simulink model "chris_3R_hsv_all_primitives_fixed_vortex"  (R2024b)
settings: Solver=FixedStepDiscrete  StartTime=0.0  StopTime=15  FixedStep=0.1  MaxStep=0.1  RelTol=1e-3
libraries: neural x102, realtime_pacer_lib x1, simulink x1
(part 1 of 6)
settings Model: Creator=RSL  LastModifiedBy=cwaight
settings SolverCC: AlgebraicLoopSolver=TrustRegion
settings DataIOCC: ReturnWorkspaceOutputs=off
settings DebuggingCC: UnconnectedInputMsg=warning  UnconnectedOutputMsg=warning  UnconnectedLineMsg=warning  ArithmeticOperatorsInVariantConditions=warning
settings ModelReferenceCC: EnableRefExpFcnMdlSchedulingChecks=on
settings SFSimCC: SimUseLocalCustomCode=off  CustomCodeUndefinedFunction=UseInterfaceOnly
settings RTWCC: RTWUseLocalCustomCode=off  GPUComputeCapability=3.5
settings CodeAppCC: StateflowObjectComments=on

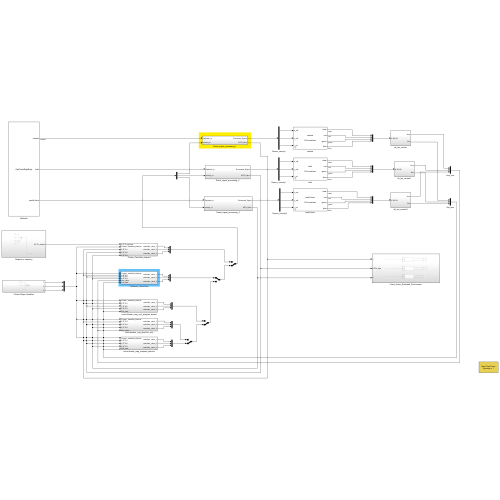
[thumbnail: Simulink's stored preview of the top-level diagram]
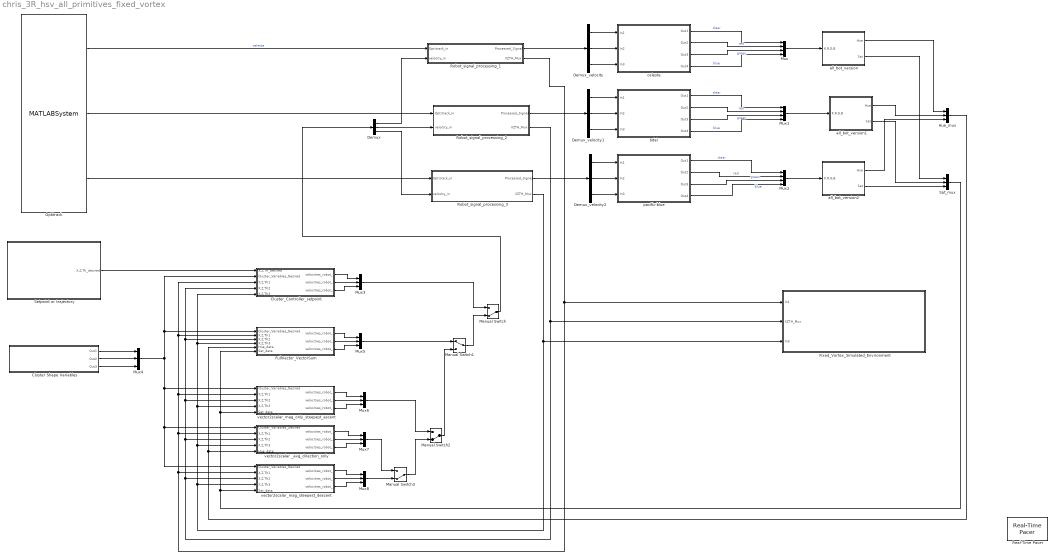
== system chris_3R_hsv_all_primitives_fixed_vortex ==
  Cluster Shape Variables : Subsystem
  Cluster_Controller_setpoint : Subsystem
  Demux : Demux  Outputs=3
  Demux_velocity : Demux  Outputs=3
  Demux_velocity1 : Demux  Outputs=3
  Demux_velocity2 : Demux  Outputs=3
  Fixed_Vortex_Simulated_Environment : Subsystem
  FullVector_VectorSum : Subsystem
  Hue_mux : Mux  Inputs=3
  Manual Switch : ManualSwitch  CurrentSetting=0
  Manual Switch1 : ManualSwitch
  Manual Switch2 : ManualSwitch  CurrentSetting=0
  Manual Switch3 : ManualSwitch  CurrentSetting=0
  Mux : Mux
  Mux1 : Mux
  Mux2 : Mux
  Mux{3..8} (6 alike) : Mux  Inputs=3
  Optitrack : MATLABSystem  System=OptiTrackRigidBody  coordinateTransformationMatrix=[ 1, 0, 0; 0, 0, 1; 0, -1, 0 ]  rigidBodyNames={ 'celeste','tidal','pacific-blue'}  orientationFormat=Euler angles  debug=on  natNetHostAddress=127.0.0.1  natNetClientAddress=127.0.0.1  dllPath=C:\DecaMATLAB\NatNetSDK\lib\x64\NatNetML.dll  unicast=off
      mask Type: OptiTrackRigidBody
      mask Display:
      | disp('OptiTrackRigidBody');
      | port_label('output',1,'celeste');
      | port_label('output',2,'tidal');
      | port_label('output',3,'pacific-blue');
  Real-Time Pacer : realtime_pacer_lib/Real-Time Pacer  simTimePerRealTime=1
  Robot_signal_processing_1 : Subsystem
  Robot_signal_processing_2 : Subsystem
  Robot_signal_processing_3 : Subsystem
  Sat_mux : Mux  Inputs=3
  Setpoint or trajectory : Subsystem
  all_bot_version : Subsystem
  all_bot_version1 : Subsystem
  all_bot_version2 : Subsystem
  celeste : Subsystem  mask(DecabotMask){robotName=celeste, decabotHelper=localhost, robotAddress=, useDataTurbine=off, useDirectSocket=on, debug=off}
      mask prompts: robotName "Robot name:"; decabotHelper "DecabotHelper/DataTurbine server:"; robotAddress "Robot network address (optional):"; useDataTurbine "Use DataTurbine"; useDirectSocket "Use direct robot TCP connection"; debug "Log debug messages"
      mask help: This is a masked subsystem that contains a Decabot block for bidirectional communication with a decabot over a direct TCP socket connection.
      mask init:
      | robotName = 'Nobody';
      | decabotHelper = 'localhost';
      | robotAddress = '';
      | useDataTurbine = true;
      | debug = true;
      mask TypeOptions robotName: decabot/robotName
      mask Callback robotName:
      | try
      |     set_param( gcb( ), 'Name', get_param( gcb( ), 'robotName' ) );
      | end
      mask TypeOptions decabotHelper: decabot/decabotHelper
      mask TypeOptions robotAddress: decabot/robotAddress
      mask TypeOptions useDataTurbine: decabot/useDataTurbine
      mask TypeOptions useDirectSocket: decabot/useDirectSocket
      mask TypeOptions debug: decabot/debug
      mask Display:
      | disp( [get_param( gcb( ), 'robotName' ) '\n\nDH: ' get_param( gcb( ), 'decabotHelper' ) ] );
      | 
      | port_label('input',1,'x_vel');
      | port_label('input',2,'y_vel');
      | port_label('input',3,'t_vel');
      | 
      | port_label('output',1,'clear');
      | port_label('output',2,'red');
      | port_label('output',3,'green');
      | port_label('output',4,'blue');
  pacific-blue : Subsystem  mask(DecabotMask){robotName=pacific-blue, decabotHelper=localhost, robotAddress=, useDataTurbine=off, useDirectSocket=on, debug=off}
      mask prompts: robotName "Robot name:"; decabotHelper "DecabotHelper/DataTurbine server:"; robotAddress "Robot network address (optional):"; useDataTurbine "Use DataTurbine"; useDirectSocket "Use direct robot TCP connection"; debug "Log debug messages"
      mask help: This is a masked subsystem that contains a Decabot block for bidirectional communication with a decabot over a direct TCP socket connection.
      mask init:
      | robotName = 'Nobody';
      | decabotHelper = 'localhost';
      | robotAddress = '';
      | useDataTurbine = true;
      | debug = true;
      mask TypeOptions robotName: decabot/robotName
      mask Callback robotName:
      | try
      |     set_param( gcb( ), 'Name', get_param( gcb( ), 'robotName' ) );
      | end
      mask TypeOptions decabotHelper: decabot/decabotHelper
      mask TypeOptions robotAddress: decabot/robotAddress
      mask TypeOptions useDataTurbine: decabot/useDataTurbine
      mask TypeOptions useDirectSocket: decabot/useDirectSocket
      mask TypeOptions debug: decabot/debug
      mask Display:
      | disp( [get_param( gcb( ), 'robotName' ) '\n\nDH: ' get_param( gcb( ), 'decabotHelper' ) ] );
      | 
      | port_label('input',1,'x_vel');
      | port_label('input',2,'y_vel');
      | port_label('input',3,'t_vel');
      | 
      | port_label('output',1,'clear');
      | port_label('output',2,'red');
      | port_label('output',3,'green');
      | port_label('output',4,'blue');
  tidal : Subsystem  mask(DecabotMask){robotName=tidal, decabotHelper=localhost, robotAddress=, useDataTurbine=off, useDirectSocket=on, debug=off}
      mask prompts: robotName "Robot name:"; decabotHelper "DecabotHelper/DataTurbine server:"; robotAddress "Robot network address (optional):"; useDataTurbine "Use DataTurbine"; useDirectSocket "Use direct robot TCP connection"; debug "Log debug messages"
      mask help: This is a masked subsystem that contains a Decabot block for bidirectional communication with a decabot over a direct TCP socket connection.
      mask init:
      | robotName = 'Nobody';
      | decabotHelper = 'localhost';
      | robotAddress = '';
      | useDataTurbine = true;
      | debug = true;
      mask TypeOptions robotName: decabot/robotName
      mask Callback robotName:
      | try
      |     set_param( gcb( ), 'Name', get_param( gcb( ), 'robotName' ) );
      | end
      mask TypeOptions decabotHelper: decabot/decabotHelper
      mask TypeOptions robotAddress: decabot/robotAddress
      mask TypeOptions useDataTurbine: decabot/useDataTurbine
      mask TypeOptions useDirectSocket: decabot/useDirectSocket
      mask TypeOptions debug: decabot/debug
      mask Display:
      | disp( [get_param( gcb( ), 'robotName' ) '\n\nDH: ' get_param( gcb( ), 'decabotHelper' ) ] );
      | 
      | port_label('input',1,'x_vel');
      | port_label('input',2,'y_vel');
      | port_label('input',3,'t_vel');
      | 
      | port_label('output',1,'clear');
      | port_label('output',2,'red');
      | port_label('output',3,'green');
      | port_label('output',4,'blue');
  vector2scalar _avg_direction_only : Subsystem
  vector2scalar_mag_only_steepest_ascent : Subsystem
  vector2scalar_mag_steepest_descent : Subsystem
  wires:
  Demux_velocity/3 -> celeste/3(In3)
  Demux_velocity/1 -> celeste/1(In1)
  Demux_velocity/2 -> celeste/2(In2)
  Optitrack/1 -> Robot_signal_processing_1/1(Optitrack_in)  "celeste"
  Robot_signal_processing_1/1(Processed_Signal) -> Demux_velocity/1
  celeste/1(Out1) -> Mux/1  "clear"
  celeste/2(Out2) -> Mux/2  "red"
  celeste/3(Out3) -> Mux/3  "green"
  celeste/4(Out4) -> Mux/4  "blue"
  Robot_signal_processing_1/2(XZTH_Mux) -> vector2scalar_mag_steepest_descent/2(X,Z,Th1), vector2scalar _avg_direction_only/2(X,Z,Th1), vector2scalar_mag_only_steepest_ascent/2(X,Z,Th1), FullVector_VectorSum/2(X,Z,Th1), Cluster_Controller_setpoint/3(X,Z,Th1), Fixed_Vortex_Simulated_Environment/1(In1)
  Mux/1 -> all_bot_version/1(K,R,G,B)
  Demux_velocity1/3 -> tidal/3(In3)
  Demux_velocity1/1 -> tidal/1(In1)
  Demux_velocity1/2 -> tidal/2(In2)
  Robot_signal_processing_2/1(Processed_Signal) -> Demux_velocity1/1
  tidal/1(Out1) -> Mux1/1  "clear"
  tidal/2(Out2) -> Mux1/2  "red"
  tidal/3(Out3) -> Mux1/3  "green"
  tidal/4(Out4) -> Mux1/4  "blue"
  Mux1/1 -> all_bot_version1/1(K,R,G,B)
  Demux_velocity2/3 -> pacific-blue/3(In3)
  Demux_velocity2/1 -> pacific-blue/1(In1)
  Demux_velocity2/2 -> pacific-blue/2(In2)
  Robot_signal_processing_3/1(Processed_Signal) -> Demux_velocity2/1
  pacific-blue/1(Out1) -> Mux2/1  "clear"
  pacific-blue/2(Out2) -> Mux2/2  "red"
  pacific-blue/3(Out3) -> Mux2/3  "green"
  pacific-blue/4(Out4) -> Mux2/4  "blue"
  Mux2/1 -> all_bot_version2/1(K,R,G,B)
  Robot_signal_processing_3/2(XZTH_Mux) -> vector2scalar_mag_steepest_descent/4(X,Z,Th3), vector2scalar _avg_direction_only/4(X,Z,Th3), vector2scalar_mag_only_steepest_ascent/4(X,Z,Th3), FullVector_VectorSum/4(X,Z,Th3), Cluster_Controller_setpoint/5(X,Z,Th3), Fixed_Vortex_Simulated_Environment/3(In3)
  Optitrack/2 -> Robot_signal_processing_2/1(Optitrack_in)
  Optitrack/3 -> Robot_signal_processing_3/1(Optitrack_in)
  Cluster_Controller_setpoint/1(velocities_robot_1) -> Mux3/1
  Cluster_Controller_setpoint/3(velocities_robot_3) -> Mux3/3
  Cluster_Controller_setpoint/2(velocities_robot_2) -> Mux3/2
  Mux4/1 -> vector2scalar_mag_only_steepest_ascent/1(Cluster_Variables_Desired), vector2scalar _avg_direction_only/1(Cluster_Variables_Desired), vector2scalar_mag_steepest_descent/1(Cluster_Variables_Desired), FullVector_VectorSum/1(Cluster_Variables_Desired), Cluster_Controller_setpoint/2(Cluster_Variables_Desired)
  Robot_signal_processing_2/2(XZTH_Mux) -> vector2scalar_mag_steepest_descent/3(X,Z,Th2), vector2scalar_mag_only_steepest_ascent/3(X,Z,Th2), FullVector_VectorSum/3(X,Z,Th2), Cluster_Controller_setpoint/4(X,Z,Th2), vector2scalar _avg_direction_only/3(X,Z,Th2), Fixed_Vortex_Simulated_Environment/2(XZTH_Mux)
  Cluster Shape Variables/1(Out1) -> Mux4/1
  Cluster Shape Variables/3(Out3) -> Mux4/3
  Setpoint or trajectory/1(X,Z,Th_desired) -> Cluster_Controller_setpoint/1(X,Z,Th_desired)
  Demux/1 -> Robot_signal_processing_1/2(velocity_in)
  Demux/2 -> Robot_signal_processing_2/2(velocity_in)
  Demux/3 -> Robot_signal_processing_3/2(velocity_in)
  Mux3/1 -> Manual Switch/1
  Manual Switch/1 -> Demux/1
  FullVector_VectorSum/1(velocities_robot_1) -> Mux5/1
  FullVector_VectorSum/2(velocities_robot_2) -> Mux5/2
  FullVector_VectorSum/3(velocities_robot_3) -> Mux5/3
  all_bot_version1/1(Hue) -> Hue_mux/2
  all_bot_version2/1(Hue) -> Hue_mux/3
  all_bot_version2/2(Sat) -> Sat_mux/3
  Hue_mux/1 -> FullVector_VectorSum/5(Hue_data), vector2scalar _avg_direction_only/5(Hue_data)
  Sat_mux/1 -> vector2scalar_mag_steepest_descent/5(Sat_data), FullVector_VectorSum/6(Sat_data), vector2scalar_mag_only_steepest_ascent/5(Sat_data)
  vector2scalar_mag_only_steepest_ascent/1(velocities_robot_1) -> Mux6/1
  vector2scalar_mag_only_steepest_ascent/2(velocities_robot_2) -> Mux6/2
  vector2scalar_mag_only_steepest_ascent/3(velocities_robot_3) -> Mux6/3
  Mux5/1 -> Manual Switch1/1
  Manual Switch1/1 -> Manual Switch/2
  all_bot_version/2(Sat) -> Sat_mux/1
  all_bot_version/1(Hue) -> Hue_mux/1
  Mux6/1 -> Manual Switch2/1
  Manual Switch2/1 -> Manual Switch1/2
  vector2scalar _avg_direction_only/1(velocities_robot_1) -> Mux7/1
  vector2scalar _avg_direction_only/2(velocities_robot_2) -> Mux7/2
  vector2scalar _avg_direction_only/3(velocities_robot_3) -> Mux7/3
  vector2scalar_mag_steepest_descent/3(velocities_robot_3) -> Mux8/3
  vector2scalar_mag_steepest_descent/2(velocities_robot_2) -> Mux8/2
  vector2scalar_mag_steepest_descent/1(velocities_robot_1) -> Mux8/1
  Mux8/1 -> Manual Switch3/2
  Mux7/1 -> Manual Switch3/1
  Manual Switch3/1 -> Manual Switch2/2
  Cluster Shape Variables/2(Out2) -> Mux4/2
  all_bot_version1/2(Sat) -> Sat_mux/2

== system chris_3R_hsv_all_primitives_fixed_vortex/Cluster Shape Variables ==
  Cluster Variable C : Constant  Value=pi/3
  Cluster_Variable_B : Constant  Value=0.35
  Cluster_variable_A : Constant  Value=0.35
  Out1 : Outport
  Out2 : Outport  Port=2
  Out3 : Outport  Port=3
  wires:
  Cluster_variable_A/1 -> Out1/1
  Cluster Variable C/1 -> Out3/1
  Cluster_Variable_B/1 -> Out2/1

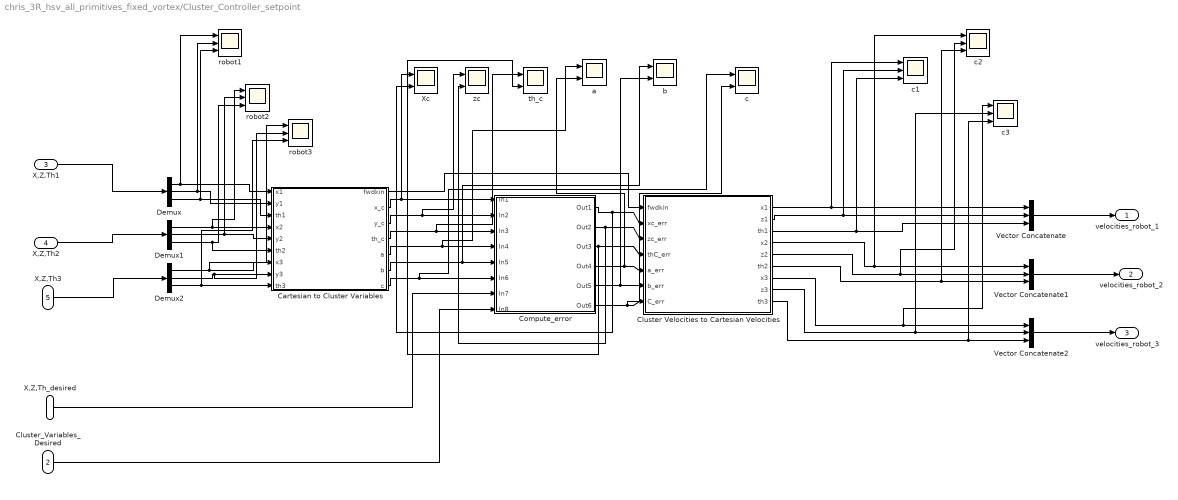
== system chris_3R_hsv_all_primitives_fixed_vortex/Cluster_Controller_setpoint ==
  X,Z,Th_desired : Inport
  Cluster_Variables_Desired : Inport  Port=2
  X,Z,Th1 : Inport  Port=3
  X,Z,Th2 : Inport  Port=4
  X,Z,Th3 : Inport  Port=5
  Cartesian to Cluster Variables : MATLAB Function  TreatAsAtomicUnit=on
  Cluster Velocities to Cartesian Velocities : MATLAB Function  TreatAsAtomicUnit=on
  Compute_error : Subsystem
  Demux : Demux  Outputs=3
  Demux1 : Demux  Outputs=3
  Demux2 : Demux  Outputs=3
  Vector Concatenate : Concatenate  NumInputs=3
  Vector Concatenate1 : Concatenate  NumInputs=3
  Vector Concatenate2 : Concatenate  NumInputs=3
  Xc : Scope  NumInputPorts=2
  a : Scope  NumInputPorts=2
  b : Scope  NumInputPorts=2
  c : Scope  NumInputPorts=2
  c1 : Scope  NumInputPorts=3
  c2 : Scope  NumInputPorts=3
  c3 : Scope  NumInputPorts=3
  robot1 : Scope  NumInputPorts=3
  robot2 : Scope  NumInputPorts=3
  robot3 : Scope  NumInputPorts=3
  th_c : Scope  NumInputPorts=2
  zc : Scope  NumInputPorts=2
  velocities_robot_1 : Outport
  velocities_robot_2 : Outport  Port=2
  velocities_robot_3 : Outport  Port=3
  wires:
  X,Z,Th1/1 -> Demux/1
  X,Z,Th2/1 -> Demux1/1
  X,Z,Th3/1 -> Demux2/1
  Vector Concatenate/1 -> velocities_robot_1/1
  Cluster Velocities to Cartesian Velocities/2(z1) -> c1/2, Vector Concatenate/2
  Cluster Velocities to Cartesian Velocities/1(x1) -> c1/1, Vector Concatenate/1
  Vector Concatenate1/1 -> velocities_robot_2/1
  Cluster Velocities to Cartesian Velocities/5(z2) -> c2/2, Vector Concatenate1/2
  Cluster Velocities to Cartesian Velocities/4(x2) -> c2/1, Vector Concatenate1/1
  Vector Concatenate2/1 -> velocities_robot_3/1
  Cluster Velocities to Cartesian Velocities/8(z3) -> c3/2, Vector Concatenate2/2
  Cluster Velocities to Cartesian Velocities/7(x3) -> c3/1, Vector Concatenate2/1
  Demux/1 -> robot1/1, Cartesian to Cluster Variables/1(x1)
  Demux/2 -> robot1/2, Cartesian to Cluster Variables/2(y1)
  Demux/3 -> robot1/3, Cartesian to Cluster Variables/3(th1)
  Demux1/1 -> robot2/1, Cartesian to Cluster Variables/4(x2)
  Demux1/2 -> robot2/2, Cartesian to Cluster Variables/5(y2)
  Demux1/3 -> robot2/3, Cartesian to Cluster Variables/6(th2)
  Demux2/1 -> robot3/1, Cartesian to Cluster Variables/7(x3)
  Demux2/2 -> robot3/2, Cartesian to Cluster Variables/8(y3)
  Demux2/3 -> robot3/3, Cartesian to Cluster Variables/9(th3)
  Cartesian to Cluster Variables/2(x_c) -> Xc/1, Compute_error/1(In1)
  Cartesian to Cluster Variables/3(y_c) -> zc/1, Compute_error/2(In2)
  Cartesian to Cluster Variables/4(th_c) -> th_c/1, Compute_error/3(In3)
  Cartesian to Cluster Variables/5(a) -> a/1, Compute_error/4(In4)
  Cartesian to Cluster Variables/6(b) -> b/1, Compute_error/5(In5)
  Cartesian to Cluster Variables/7(c) -> c/1, Compute_error/6(In6)
  X,Z,Th_desired/1 -> Compute_error/7(In7)
  Cluster_Variables_Desired/1 -> Compute_error/8(In8)
  Compute_error/1(Out1) -> Xc/2, Cluster Velocities to Cartesian Velocities/2(xc_err)
  Compute_error/2(Out2) -> zc/2, Cluster Velocities to Cartesian Velocities/3(zc_err)
  Compute_error/3(Out3) -> th_c/2, Cluster Velocities to Cartesian Velocities/4(thC_err)
  Compute_error/4(Out4) -> a/2, Cluster Velocities to Cartesian Velocities/5(a_err)
  Compute_error/5(Out5) -> b/2, Cluster Velocities to Cartesian Velocities/6(b_err)
  Compute_error/6(Out6) -> c/2, Cluster Velocities to Cartesian Velocities/7(C_err)
  Cartesian to Cluster Variables/1(fwdkin) -> Cluster Velocities to Cartesian Velocities/1(fwdkin)
  Cluster Velocities to Cartesian Velocities/3(th1) -> c1/3, Vector Concatenate/3
  Cluster Velocities to Cartesian Velocities/6(th2) -> c2/3, Vector Concatenate1/3
  Cluster Velocities to Cartesian Velocities/9(th3) -> c3/3, Vector Concatenate2/3

== system chris_3R_hsv_all_primitives_fixed_vortex/Fixed_Vortex_Simulated_Environment ==
  In1 : Inport
  XZTH_Mux : Inport  Port=2
  In3 : Inport  Port=3
  Demux_velocity1 : Demux  Outputs=3
  Demux_velocity2 : Demux  Outputs=3
  Demux_velocity3 : Demux  Outputs=3
  Fixed_Vortex_Simulator : MATLAB Function  TreatAsAtomicUnit=on
  Fixed_Vortex_Simulator1 : MATLAB Function  TreatAsAtomicUnit=on
  Fixed_Vortex_Simulator2 : MATLAB Function  TreatAsAtomicUnit=on
  To Workspace1 : ToWorkspace  VariableName=hue_anticipated1  SampleTime=-1
  To Workspace2 : ToWorkspace  VariableName=sat_anticipated1  SampleTime=-1
  To Workspace3 : ToWorkspace  VariableName=hue_anticipated2  SampleTime=-1
  To Workspace4 : ToWorkspace  VariableName=sat_anticipated2  SampleTime=-1
  To Workspace5 : ToWorkspace  VariableName=hue_anticipated3  SampleTime=-1
  To Workspace6 : ToWorkspace  VariableName=sat_anticipated3  SampleTime=-1
  wires:
  Demux_velocity3/2 -> Fixed_Vortex_Simulator/2(z)
  Demux_velocity3/3 -> Fixed_Vortex_Simulator/3(th)
  Demux_velocity3/1 -> Fixed_Vortex_Simulator/1(x)
  Fixed_Vortex_Simulator/2(sat_anticipated) -> To Workspace2/1
  Fixed_Vortex_Simulator/1(hue_anticipated) -> To Workspace1/1
  In1/1 -> Demux_velocity3/1
  Fixed_Vortex_Simulator1/1(hue_anticipated) -> To Workspace3/1
  Demux_velocity1/3 -> Fixed_Vortex_Simulator1/3(th)
  Demux_velocity1/1 -> Fixed_Vortex_Simulator1/1(x)
  Fixed_Vortex_Simulator1/2(sat_anticipated) -> To Workspace4/1
  XZTH_Mux/1 -> Demux_velocity1/1
  Demux_velocity1/2 -> Fixed_Vortex_Simulator1/2(z)
  Fixed_Vortex_Simulator2/1(hue_anticipated) -> To Workspace5/1
  Demux_velocity2/3 -> Fixed_Vortex_Simulator2/3(th)
  Demux_velocity2/1 -> Fixed_Vortex_Simulator2/1(x)
  Fixed_Vortex_Simulator2/2(sat_anticipated) -> To Workspace6/1
  In3/1 -> Demux_velocity2/1
  Demux_velocity2/2 -> Fixed_Vortex_Simulator2/2(z)

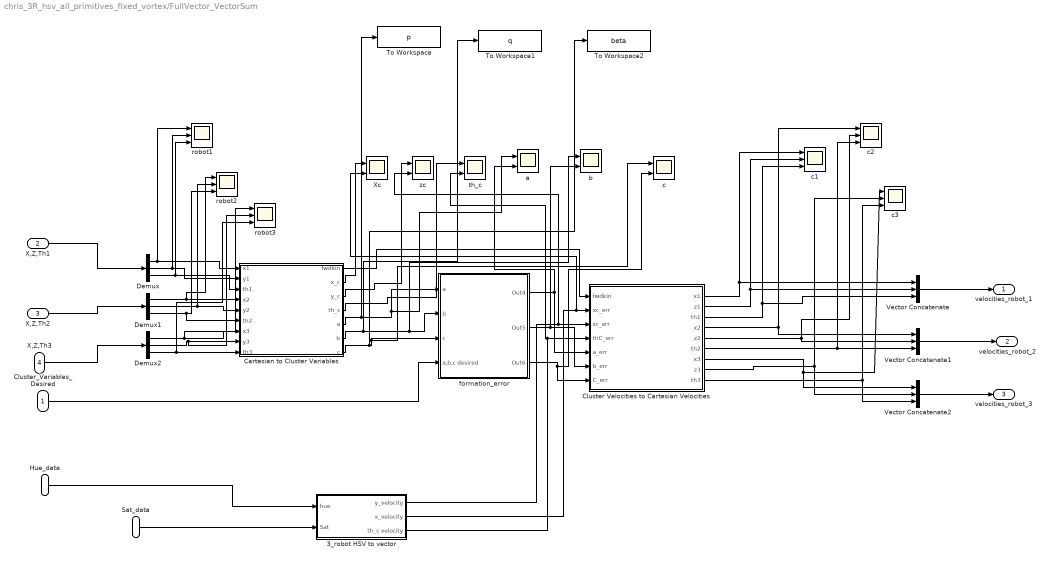
== system chris_3R_hsv_all_primitives_fixed_vortex/FullVector_VectorSum ==
  Cluster_Variables_Desired : Inport
  X,Z,Th1 : Inport  Port=2
  X,Z,Th2 : Inport  Port=3
  X,Z,Th3 : Inport  Port=4
  Hue_data : Inport  Port=5
  Sat_data : Inport  Port=6
  3_robot HSV to vector : Subsystem
  Cartesian to Cluster Variables : MATLAB Function  TreatAsAtomicUnit=on
  Cluster Velocities to Cartesian Velocities : MATLAB Function  TreatAsAtomicUnit=on
  Demux : Demux  Outputs=3
  Demux1 : Demux  Outputs=3
  Demux2 : Demux  Outputs=3
  To Workspace : ToWorkspace  VariableName=p  SampleTime=-1
  To Workspace1 : ToWorkspace  VariableName=q  SampleTime=-1
  To Workspace2 : ToWorkspace  VariableName=beta  SampleTime=-1
  Vector Concatenate : Concatenate  NumInputs=3
  Vector Concatenate1 : Concatenate  NumInputs=3
  Vector Concatenate2 : Concatenate  NumInputs=3
  Xc : Scope  NumInputPorts=2
  a : Scope  NumInputPorts=2
  b : Scope  NumInputPorts=2
  c : Scope  NumInputPorts=2
  c1 : Scope  NumInputPorts=3
  c2 : Scope  NumInputPorts=3
  c3 : Scope  NumInputPorts=3
  formation_error : Subsystem
  robot1 : Scope  NumInputPorts=3
  robot2 : Scope  NumInputPorts=3
  robot3 : Scope  NumInputPorts=3
  th_c : Scope  NumInputPorts=2
  zc : Scope  NumInputPorts=2
  velocities_robot_1 : Outport
  velocities_robot_2 : Outport  Port=2
  velocities_robot_3 : Outport  Port=3
  wires:
  X,Z,Th1/1 -> Demux/1
  X,Z,Th2/1 -> Demux1/1
  X,Z,Th3/1 -> Demux2/1
  Vector Concatenate/1 -> velocities_robot_1/1
  Cluster Velocities to Cartesian Velocities/2(z1) -> c1/2, Vector Concatenate/2
  Cluster Velocities to Cartesian Velocities/1(x1) -> c1/1, Vector Concatenate/1
  Vector Concatenate1/1 -> velocities_robot_2/1
  Cluster Velocities to Cartesian Velocities/5(z2) -> c2/2, Vector Concatenate1/2
  Cluster Velocities to Cartesian Velocities/4(x2) -> c2/1, Vector Concatenate1/1
  Vector Concatenate2/1 -> velocities_robot_3/1
  Cluster Velocities to Cartesian Velocities/8(z3) -> c3/2, Vector Concatenate2/2
  Cluster Velocities to Cartesian Velocities/7(x3) -> Vector Concatenate2/1, c3/1
  Demux/1 -> robot1/1, Cartesian to Cluster Variables/1(x1)
  Demux/2 -> robot1/2, Cartesian to Cluster Variables/2(y1)
  Demux/3 -> robot1/3, Cartesian to Cluster Variables/3(th1)
  Demux1/1 -> robot2/1, Cartesian to Cluster Variables/4(x2)
  Demux1/2 -> robot2/2, Cartesian to Cluster Variables/5(y2)
  Demux1/3 -> robot2/3, Cartesian to Cluster Variables/6(th2)
  Demux2/1 -> robot3/1, Cartesian to Cluster Variables/7(x3)
  Demux2/2 -> robot3/2, Cartesian to Cluster Variables/8(y3)
  Demux2/3 -> robot3/3, Cartesian to Cluster Variables/9(th3)
  Cartesian to Cluster Variables/2(x_c) -> Xc/1
  Cartesian to Cluster Variables/3(y_c) -> zc/1
  Cartesian to Cluster Variables/4(th_c) -> th_c/1
  Cartesian to Cluster Variables/5(a) -> To Workspace/1, a/1, formation_error/1(a)
  Cartesian to Cluster Variables/6(b) -> To Workspace1/1, b/1, formation_error/2(b)
  Cartesian to Cluster Variables/7(c) -> To Workspace2/1, c/1, formation_error/3(c)
  Cluster_Variables_Desired/1 -> formation_error/4(a,b,c desired)
  formation_error/1(Out4) -> a/2, Cluster Velocities to Cartesian Velocities/5(a_err)
  formation_error/2(Out5) -> b/2, Cluster Velocities to Cartesian Velocities/6(b_err)
  formation_error/3(Out6) -> Cluster Velocities to Cartesian Velocities/7(C_err), c/2
  Cartesian to Cluster Variables/1(fwdkin) -> Cluster Velocities to Cartesian Velocities/1(fwdkin)
  Cluster Velocities to Cartesian Velocities/3(th1) -> c1/3, Vector Concatenate/3
  Cluster Velocities to Cartesian Velocities/6(th2) -> c2/3, Vector Concatenate1/3
  Cluster Velocities to Cartesian Velocities/9(th3) -> c3/3, Vector Concatenate2/3
  Hue_data/1 -> 3_robot HSV to vector/1(hue)
  Sat_data/1 -> 3_robot HSV to vector/2(Sat)
  3_robot HSV to vector/2(x_velocity) -> Xc/2, Cluster Velocities to Cartesian Velocities/2(xc_err)
  3_robot HSV to vector/1(y_velocity) -> Cluster Velocities to Cartesian Velocities/3(zc_err), zc/2
  3_robot HSV to vector/3(th_c velocity) -> Cluster Velocities to Cartesian Velocities/4(thC_err), th_c/2

== system chris_3R_hsv_all_primitives_fixed_vortex/Robot_signal_processing_1 ==
  Optitrack_in : Inport
  velocity_in : Inport  Port=2
  Demux4 : Demux  Outputs=3
  Global to Body Velocities : Product  Multiplication=Matrix(*)
  Global to Body Rotation Matrix : MATLAB Function  TreatAsAtomicUnit=on
  Math Function : Math  Operator=transpose  SignedPower=on
  Signal_Reshape : Reshape  OutputDimensions=6
  Signal_Select : Selector  InputPortWidth=6  IndexOptions=Index vector (dialog)  Indices=[1 2 6]  OutputSizes=1
  To Workspace : ToWorkspace  VariableName=robot1_pose  SampleTime=-1
  Processed_Signal : Outport
  XZTH_Mux : Outport  Port=2
  wires:
  Demux4/3 -> Global to Body Rotation Matrix/1(u)  "theta"
  Global to Body Velocities/1 -> Processed_Signal/1
  Signal_Reshape/1 -> Signal_Select/1
  velocity_in/1 -> Global to Body Velocities/2
  Optitrack_in/1 -> Signal_Reshape/1
  Global to Body Rotation Matrix/1(y) -> Math Function/1
  Math Function/1 -> Global to Body Velocities/1
  Signal_Select/1 -> To Workspace/1, XZTH_Mux/1, Demux4/1

== system chris_3R_hsv_all_primitives_fixed_vortex/Robot_signal_processing_2 ==
  Optitrack_in : Inport
  velocity_in : Inport  Port=2
  Demux4 : Demux  Outputs=3
  Global to Body Velocities : Product  Multiplication=Matrix(*)
  Global to Body Rotation Matrix : MATLAB Function  TreatAsAtomicUnit=on
  Math Function : Math  Operator=transpose  SignedPower=on
  Mux : Mux  Inputs=3
  Signal_Reshape : Reshape  OutputDimensions=6
  Signal_Select : Selector  InputPortWidth=6  IndexOptions=Index vector (dialog)  Indices=[1 2 6]  OutputSizes=1
  To Workspace : ToWorkspace  VariableName=robot2_pose  SampleTime=-1
  Processed_Signal : Outport
  XZTH_Mux : Outport  Port=2
  wires:
  Demux4/1 -> Mux/1  "X"
  Demux4/3 -> Mux/3, Global to Body Rotation Matrix/1(u)  "theta"
  Demux4/2 -> Mux/2  "Z"
  Global to Body Velocities/1 -> Processed_Signal/1
  Signal_Reshape/1 -> Signal_Select/1
  velocity_in/1 -> Global to Body Velocities/2
  Optitrack_in/1 -> Signal_Reshape/1
  Global to Body Rotation Matrix/1(y) -> Math Function/1
  Signal_Select/1 -> To Workspace/1, Demux4/1
  Math Function/1 -> Global to Body Velocities/1
  Mux/1 -> XZTH_Mux/1

== system chris_3R_hsv_all_primitives_fixed_vortex/Robot_signal_processing_3 ==
  Optitrack_in : Inport
  velocity_in : Inport  Port=2
  Demux4 : Demux  Outputs=3
  Global to Body Velocities : Product  Multiplication=Matrix(*)
  Global to Body Rotation Matrix : MATLAB Function  TreatAsAtomicUnit=on
  Math Function : Math  Operator=transpose  SignedPower=on
  Mux : Mux  Inputs=3
  Signal_Reshape : Reshape  OutputDimensions=6
  Signal_Select : Selector  InputPortWidth=6  IndexOptions=Index vector (dialog)  Indices=[1 2 6]  OutputSizes=1
  To Workspace : ToWorkspace  VariableName=robot3_pose  SampleTime=-1
  Processed_Signal : Outport
  XZTH_Mux : Outport  Port=2
  wires:
  Demux4/1 -> Mux/1  "X"
  Demux4/3 -> Mux/3, Global to Body Rotation Matrix/1(u)  "theta"
  Demux4/2 -> Mux/2  "Z"
  Global to Body Velocities/1 -> Processed_Signal/1
  Signal_Reshape/1 -> Signal_Select/1
  velocity_in/1 -> Global to Body Velocities/2
  Optitrack_in/1 -> Signal_Reshape/1
  Global to Body Rotation Matrix/1(y) -> Math Function/1
  Signal_Select/1 -> Demux4/1
  Math Function/1 -> Global to Body Velocities/1
  Mux/1 -> To Workspace/1, XZTH_Mux/1

== system chris_3R_hsv_all_primitives_fixed_vortex/Setpoint or trajectory ==
  Manual Switch : ManualSwitch  CurrentSetting=0
  Mux3 : Mux  Inputs=3
  Ramp : simulink/Sources/Ramp  slope=1  start=0  InitialOutput=0.1
  "Theta_Set Point1 " : Constant  Value=0.1
  X_Set Point : Constant  Value=1.5
  Z_Set Point1 : Constant  Value=0.5
  X,Z,Th_desired : Outport
  wires:
  Mux3/1 -> X,Z,Th_desired/1
  Z_Set Point1/1 -> Mux3/2
  Manual Switch/1 -> Mux3/3
  "Theta_Set Point1 "/1 -> Manual Switch/1
  X_Set Point/1 -> Mux3/1
  Ramp/1 -> Manual Switch/2

== system chris_3R_hsv_all_primitives_fixed_vortex/all_bot_version ==
  K,R,G,B : Inport
  Demux : Demux  Outputs=2
  Demux1 : Demux
  Mux : Mux  Inputs=7
  RGB to HSV : MATLAB Function  TreatAsAtomicUnit=on
  everything_hue_net : Subsystem
      mask help: Feed-Forward Neural Network
      mask Display: e = 0.06;c1 = [120 150 230]/255;c2 = ([120 150 230]+0)/383;c3 = ([120 150 230]+128)/383;patch([0 1 1 0],[0 0 1 1],c1);patch([0 1 1 1-e 1-e 0+e],[0 0 1 1-e 0+e 0+e],c2);patch([0 0 1 1-e 0+e 0+e],[0 1 1 1-e 1-e 0+e],c3);plot([0 1 1 0 0],[0 0 1 1 0]);fprintf('NNET');port_label('input',1,' Input');port_label('output',1,'Output ');
  everything_sat_net : Subsystem
      mask help: Feed-Forward Neural Network
      mask Display: e = 0.06;c1 = [120 150 230]/255;c2 = ([120 150 230]+0)/383;c3 = ([120 150 230]+128)/383;patch([0 1 1 0],[0 0 1 1],c1);patch([0 1 1 1-e 1-e 0+e],[0 0 1 1-e 0+e 0+e],c2);patch([0 0 1 1-e 0+e 0+e],[0 1 1 1-e 1-e 0+e],c3);plot([0 1 1 0 0],[0 0 1 1 0]);fprintf('NNET');port_label('input',1,' Input');port_label('output',1,'Output ');
  hue_post_processor : MATLAB Function  TreatAsAtomicUnit=on
  sat_post_processor : MATLAB Function  TreatAsAtomicUnit=on
  sat_post_processor1 : MATLAB Function  TreatAsAtomicUnit=on
  Hue : Outport
  Sat : Outport  Port=2
  wires:
  K,R,G,B/1 -> Demux1/1
  RGB to HSV/2(G) -> Mux/2
  RGB to HSV/6(S) -> Mux/6
  Mux/1 -> sat_post_processor1/1(data_raw)
  sat_post_processor/1(sat) -> Sat/1
  everything_sat_net/1(Output) -> sat_post_processor/1(sat_nn_output)
  Demux/1 -> hue_post_processor/1(hue_nn_sin)
  RGB to HSV/3(B) -> Mux/3
  RGB to HSV/7(V) -> Mux/7
  everything_hue_net/1(Output) -> Demux/1
  Demux/2 -> hue_post_processor/2(hue_nn_cos)
  hue_post_processor/1(hue) -> Hue/1
  RGB to HSV/1(R) -> Mux/1
  RGB to HSV/5(H) -> Mux/5
  RGB to HSV/4(K) -> Mux/4
  sat_post_processor1/1(data) -> everything_sat_net/1(Input), everything_hue_net/1(Input)
  Demux1/1 -> RGB to HSV/4("K ")
  Demux1/2 -> RGB to HSV/1("R ")
  Demux1/3 -> RGB to HSV/2("G ")
  Demux1/4 -> RGB to HSV/3("B ")

== system chris_3R_hsv_all_primitives_fixed_vortex/all_bot_version1 ==
  K,R,G,B : Inport
  Demux : Demux  Outputs=2
  Demux1 : Demux
  Mux : Mux  Inputs=7
  RGB to HSV : MATLAB Function  TreatAsAtomicUnit=on
  everything_hue_net : Subsystem
      mask help: Feed-Forward Neural Network
      mask Display: e = 0.06;c1 = [120 150 230]/255;c2 = ([120 150 230]+0)/383;c3 = ([120 150 230]+128)/383;patch([0 1 1 0],[0 0 1 1],c1);patch([0 1 1 1-e 1-e 0+e],[0 0 1 1-e 0+e 0+e],c2);patch([0 0 1 1-e 0+e 0+e],[0 1 1 1-e 1-e 0+e],c3);plot([0 1 1 0 0],[0 0 1 1 0]);fprintf('NNET');port_label('input',1,' Input');port_label('output',1,'Output ');
  everything_sat_net : Subsystem
      mask help: Feed-Forward Neural Network
      mask Display: e = 0.06;c1 = [120 150 230]/255;c2 = ([120 150 230]+0)/383;c3 = ([120 150 230]+128)/383;patch([0 1 1 0],[0 0 1 1],c1);patch([0 1 1 1-e 1-e 0+e],[0 0 1 1-e 0+e 0+e],c2);patch([0 0 1 1-e 0+e 0+e],[0 1 1 1-e 1-e 0+e],c3);plot([0 1 1 0 0],[0 0 1 1 0]);fprintf('NNET');port_label('input',1,' Input');port_label('output',1,'Output ');
  hue_post_processor : MATLAB Function  TreatAsAtomicUnit=on
  sat_post_processor : MATLAB Function  TreatAsAtomicUnit=on
  sat_post_processor1 : MATLAB Function  TreatAsAtomicUnit=on
  Hue : Outport
  Sat : Outport  Port=2
  wires:
  K,R,G,B/1 -> Demux1/1
  RGB to HSV/2(G) -> Mux/2
  RGB to HSV/6(S) -> Mux/6
  Mux/1 -> sat_post_processor1/1(data_raw)
  sat_post_processor/1(sat) -> Sat/1
  everything_sat_net/1(Output) -> sat_post_processor/1(sat_nn_output)
  Demux/1 -> hue_post_processor/1(hue_nn_sin)
  RGB to HSV/3(B) -> Mux/3
  RGB to HSV/7(V) -> Mux/7
  everything_hue_net/1(Output) -> Demux/1
  Demux/2 -> hue_post_processor/2(hue_nn_cos)
  hue_post_processor/1(hue) -> Hue/1
  RGB to HSV/1(R) -> Mux/1
  RGB to HSV/5(H) -> Mux/5
  RGB to HSV/4(K) -> Mux/4
  sat_post_processor1/1(data) -> everything_sat_net/1(Input), everything_hue_net/1(Input)
  Demux1/1 -> RGB to HSV/4("K ")
  Demux1/2 -> RGB to HSV/1("R ")
  Demux1/3 -> RGB to HSV/2("G ")
  Demux1/4 -> RGB to HSV/3("B ")

== system chris_3R_hsv_all_primitives_fixed_vortex/all_bot_version2 ==
  K,R,G,B : Inport
  Demux : Demux  Outputs=2
  Demux1 : Demux
  Mux : Mux  Inputs=7
  RGB to HSV : MATLAB Function  TreatAsAtomicUnit=on
  everything_hue_net : Subsystem
      mask help: Feed-Forward Neural Network
      mask Display: e = 0.06;c1 = [120 150 230]/255;c2 = ([120 150 230]+0)/383;c3 = ([120 150 230]+128)/383;patch([0 1 1 0],[0 0 1 1],c1);patch([0 1 1 1-e 1-e 0+e],[0 0 1 1-e 0+e 0+e],c2);patch([0 0 1 1-e 0+e 0+e],[0 1 1 1-e 1-e 0+e],c3);plot([0 1 1 0 0],[0 0 1 1 0]);fprintf('NNET');port_label('input',1,' Input');port_label('output',1,'Output ');
  everything_sat_net : Subsystem
      mask help: Feed-Forward Neural Network
      mask Display: e = 0.06;c1 = [120 150 230]/255;c2 = ([120 150 230]+0)/383;c3 = ([120 150 230]+128)/383;patch([0 1 1 0],[0 0 1 1],c1);patch([0 1 1 1-e 1-e 0+e],[0 0 1 1-e 0+e 0+e],c2);patch([0 0 1 1-e 0+e 0+e],[0 1 1 1-e 1-e 0+e],c3);plot([0 1 1 0 0],[0 0 1 1 0]);fprintf('NNET');port_label('input',1,' Input');port_label('output',1,'Output ');
  hue_post_processor : MATLAB Function  TreatAsAtomicUnit=on
  sat_post_processor : MATLAB Function  TreatAsAtomicUnit=on
  sat_post_processor1 : MATLAB Function  TreatAsAtomicUnit=on
  Hue : Outport
  Sat : Outport  Port=2
  wires:
  K,R,G,B/1 -> Demux1/1
  RGB to HSV/2(G) -> Mux/2
  RGB to HSV/6(S) -> Mux/6
  Mux/1 -> sat_post_processor1/1(data_raw)
  sat_post_processor/1(sat) -> Sat/1
  everything_sat_net/1(Output) -> sat_post_processor/1(sat_nn_output)
  Demux/1 -> hue_post_processor/1(hue_nn_sin)
  RGB to HSV/3(B) -> Mux/3
  RGB to HSV/7(V) -> Mux/7
  everything_hue_net/1(Output) -> Demux/1
  Demux/2 -> hue_post_processor/2(hue_nn_cos)
  hue_post_processor/1(hue) -> Hue/1
  RGB to HSV/1(R) -> Mux/1
  RGB to HSV/5(H) -> Mux/5
  RGB to HSV/4(K) -> Mux/4
  sat_post_processor1/1(data) -> everything_sat_net/1(Input), everything_hue_net/1(Input)
  Demux1/1 -> RGB to HSV/4("K ")
  Demux1/2 -> RGB to HSV/1("R ")
  Demux1/3 -> RGB to HSV/2("G ")
  Demux1/4 -> RGB to HSV/3("B ")

== system chris_3R_hsv_all_primitives_fixed_vortex/celeste ==
  In1 : Inport
  In2 : Inport  Port=2
  In3 : Inport  Port=3
  Signal Specification : SignalSpecification  OutDataTypeStr=double  Dimensions=1
  Signal Specification1 : SignalSpecification  OutDataTypeStr=double  Dimensions=1
  Signal Specification2 : SignalSpecification  OutDataTypeStr=double  Dimensions=1
  decabot : MATLABSystem  System=Decabot  robotName=celeste  decabotHelper=localhost  useDataTurbine=off  useDirectSocket=on  debug=off
      mask Type: Decabot
      mask Display:
      | disp('celeste\n\nDH: localhost');
      | port_label('input',1,'x_vel');
      | port_label('input',2,'y_vel');
      | port_label('input',3,'t_vel');
      | port_label('output',1,'clear');
      | port_label('output',2,'red');
      | port_label('output',3,'green');
      | port_label('output',4,'blue');
  Out1 : Outport
  Out2 : Outport  Port=2
  Out3 : Outport  Port=3
  Out4 : Outport  Port=4
  wires:
  Signal Specification2/1 -> decabot/3
  Signal Specification1/1 -> decabot/2
  Signal Specification/1 -> decabot/1
  In2/1 -> Signal Specification1/1
  decabot/4 -> Out4/1
  decabot/1 -> Out1/1
  decabot/3 -> Out3/1
  decabot/2 -> Out2/1
  In1/1 -> Signal Specification/1
  In3/1 -> Signal Specification2/1

== system chris_3R_hsv_all_primitives_fixed_vortex/pacific-blue ==
  In1 : Inport
  In2 : Inport  Port=2
  In3 : Inport  Port=3
  Signal Specification : SignalSpecification  OutDataTypeStr=double  Dimensions=1
  Signal Specification1 : SignalSpecification  OutDataTypeStr=double  Dimensions=1
  Signal Specification2 : SignalSpecification  OutDataTypeStr=double  Dimensions=1
  decabot : MATLABSystem  System=Decabot  robotName=pacific-blue  decabotHelper=localhost  useDataTurbine=off  useDirectSocket=on  debug=off
      mask Type: Decabot
      mask Display:
      | disp('pacific-blue\n\nDH: localhost');
      | port_label('input',1,'x_vel');
      | port_label('input',2,'y_vel');
      | port_label('input',3,'t_vel');
      | port_label('output',1,'clear');
      | port_label('output',2,'red');
      | port_label('output',3,'green');
      | port_label('output',4,'blue');
  Out1 : Outport
  Out2 : Outport  Port=2
  Out3 : Outport  Port=3
  Out4 : Outport  Port=4
  wires:
  Signal Specification2/1 -> decabot/3
  Signal Specification1/1 -> decabot/2
  Signal Specification/1 -> decabot/1
  In2/1 -> Signal Specification1/1
  decabot/4 -> Out4/1
  decabot/1 -> Out1/1
  decabot/3 -> Out3/1
  decabot/2 -> Out2/1
  In1/1 -> Signal Specification/1
  In3/1 -> Signal Specification2/1

== system chris_3R_hsv_all_primitives_fixed_vortex/tidal ==
  In1 : Inport
  In2 : Inport  Port=2
  In3 : Inport  Port=3
  Signal Specification : SignalSpecification  OutDataTypeStr=double  Dimensions=1
  Signal Specification1 : SignalSpecification  OutDataTypeStr=double  Dimensions=1
  Signal Specification2 : SignalSpecification  OutDataTypeStr=double  Dimensions=1
  decabot : MATLABSystem  System=Decabot  robotName=tidal  decabotHelper=localhost  useDataTurbine=off  useDirectSocket=on  debug=off
      mask Type: Decabot
      mask Display:
      | disp('tidal\n\nDH: localhost');
      | port_label('input',1,'x_vel');
      | port_label('input',2,'y_vel');
      | port_label('input',3,'t_vel');
      | port_label('output',1,'clear');
      | port_label('output',2,'red');
      | port_label('output',3,'green');
      | port_label('output',4,'blue');
  Out1 : Outport
  Out2 : Outport  Port=2
  Out3 : Outport  Port=3
  Out4 : Outport  Port=4
  wires:
  Signal Specification2/1 -> decabot/3
  Signal Specification1/1 -> decabot/2
  Signal Specification/1 -> decabot/1
  In2/1 -> Signal Specification1/1
  decabot/4 -> Out4/1
  decabot/1 -> Out1/1
  decabot/3 -> Out3/1
  decabot/2 -> Out2/1
  In1/1 -> Signal Specification/1
  In3/1 -> Signal Specification2/1

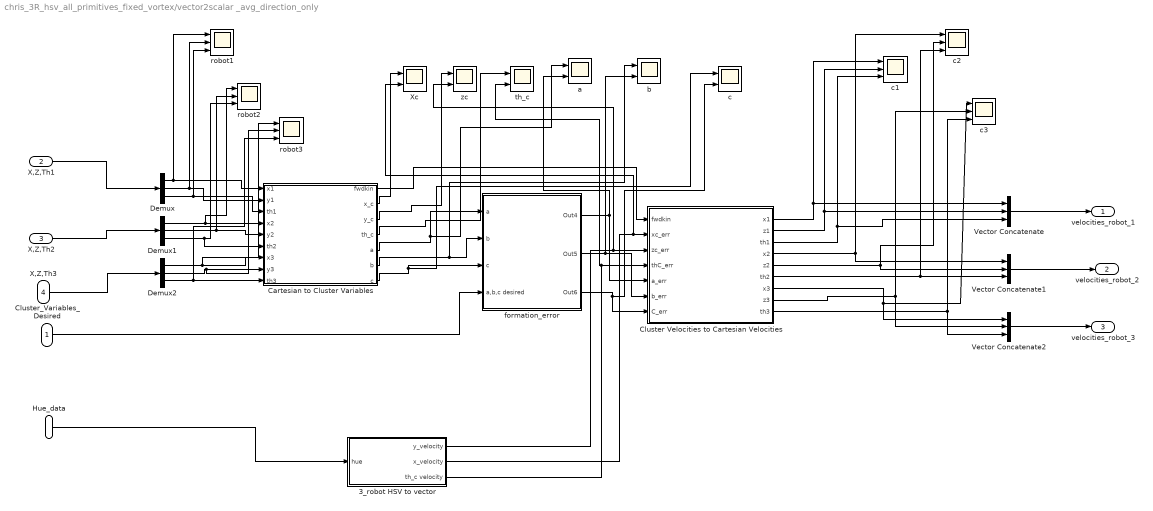
== system chris_3R_hsv_all_primitives_fixed_vortex/vector2scalar _avg_direction_only ==
  Cluster_Variables_Desired : Inport
  X,Z,Th1 : Inport  Port=2
  X,Z,Th2 : Inport  Port=3
  X,Z,Th3 : Inport  Port=4
  Hue_data : Inport  Port=5
  3_robot HSV to vector : Subsystem
  Cartesian to Cluster Variables : MATLAB Function  TreatAsAtomicUnit=on
  Cluster Velocities to Cartesian Velocities : MATLAB Function  TreatAsAtomicUnit=on
  Demux : Demux  Outputs=3
  Demux1 : Demux  Outputs=3
  Demux2 : Demux  Outputs=3
  Vector Concatenate : Concatenate  NumInputs=3
  Vector Concatenate1 : Concatenate  NumInputs=3
  Vector Concatenate2 : Concatenate  NumInputs=3
  Xc : Scope  NumInputPorts=2
  a : Scope  NumInputPorts=2
  b : Scope  NumInputPorts=2
  c : Scope  NumInputPorts=2
  c1 : Scope  NumInputPorts=3
  c2 : Scope  NumInputPorts=3
  c3 : Scope  NumInputPorts=3
  formation_error : Subsystem
  robot1 : Scope  NumInputPorts=3
  robot2 : Scope  NumInputPorts=3
  robot3 : Scope  NumInputPorts=3
  th_c : Scope  NumInputPorts=2
  zc : Scope  NumInputPorts=2
  velocities_robot_1 : Outport
  velocities_robot_2 : Outport  Port=2
  velocities_robot_3 : Outport  Port=3
  wires:
  X,Z,Th1/1 -> Demux/1
  X,Z,Th2/1 -> Demux1/1
  X,Z,Th3/1 -> Demux2/1
  Vector Concatenate/1 -> velocities_robot_1/1
  Cluster Velocities to Cartesian Velocities/2(z1) -> c1/2, Vector Concatenate/2
  Cluster Velocities to Cartesian Velocities/1(x1) -> c1/1, Vector Concatenate/1
  Vector Concatenate1/1 -> velocities_robot_2/1
  Cluster Velocities to Cartesian Velocities/5(z2) -> c2/2, Vector Concatenate1/2
  Cluster Velocities to Cartesian Velocities/4(x2) -> c2/1, Vector Concatenate1/1
  Vector Concatenate2/1 -> velocities_robot_3/1
  Cluster Velocities to Cartesian Velocities/8(z3) -> c3/2, Vector Concatenate2/2
  Cluster Velocities to Cartesian Velocities/7(x3) -> Vector Concatenate2/1, c3/1
  Demux/1 -> robot1/1, Cartesian to Cluster Variables/1(x1)
  Demux/2 -> robot1/2, Cartesian to Cluster Variables/2(y1)
  Demux/3 -> robot1/3, Cartesian to Cluster Variables/3(th1)
  Demux1/1 -> robot2/1, Cartesian to Cluster Variables/4(x2)
  Demux1/2 -> robot2/2, Cartesian to Cluster Variables/5(y2)
  Demux1/3 -> robot2/3, Cartesian to Cluster Variables/6(th2)
  Demux2/1 -> robot3/1, Cartesian to Cluster Variables/7(x3)
  Demux2/2 -> robot3/2, Cartesian to Cluster Variables/8(y3)
  Demux2/3 -> robot3/3, Cartesian to Cluster Variables/9(th3)
  Cartesian to Cluster Variables/2(x_c) -> Xc/1
  Cartesian to Cluster Variables/3(y_c) -> zc/1
  Cartesian to Cluster Variables/4(th_c) -> th_c/1
  Cartesian to Cluster Variables/5(a) -> a/1, formation_error/1(a)
  Cartesian to Cluster Variables/6(b) -> b/1, formation_error/2(b)
  Cartesian to Cluster Variables/7(c) -> c/1, formation_error/3(c)
  Cluster_Variables_Desired/1 -> formation_error/4(a,b,c desired)
  formation_error/1(Out4) -> a/2, Cluster Velocities to Cartesian Velocities/5(a_err)
  formation_error/2(Out5) -> b/2, Cluster Velocities to Cartesian Velocities/6(b_err)
  formation_error/3(Out6) -> Cluster Velocities to Cartesian Velocities/7(C_err), c/2
  Cartesian to Cluster Variables/1(fwdkin) -> Cluster Velocities to Cartesian Velocities/1(fwdkin)
  Cluster Velocities to Cartesian Velocities/3(th1) -> c1/3, Vector Concatenate/3
  Cluster Velocities to Cartesian Velocities/6(th2) -> c2/3, Vector Concatenate1/3
  Cluster Velocities to Cartesian Velocities/9(th3) -> c3/3, Vector Concatenate2/3
  Hue_data/1 -> 3_robot HSV to vector/1(hue)
  3_robot HSV to vector/2(x_velocity) -> Xc/2, Cluster Velocities to Cartesian Velocities/2(xc_err)
  3_robot HSV to vector/1(y_velocity) -> Cluster Velocities to Cartesian Velocities/3(zc_err), zc/2
  3_robot HSV to vector/3(th_c velocity) -> Cluster Velocities to Cartesian Velocities/4(thC_err), th_c/2

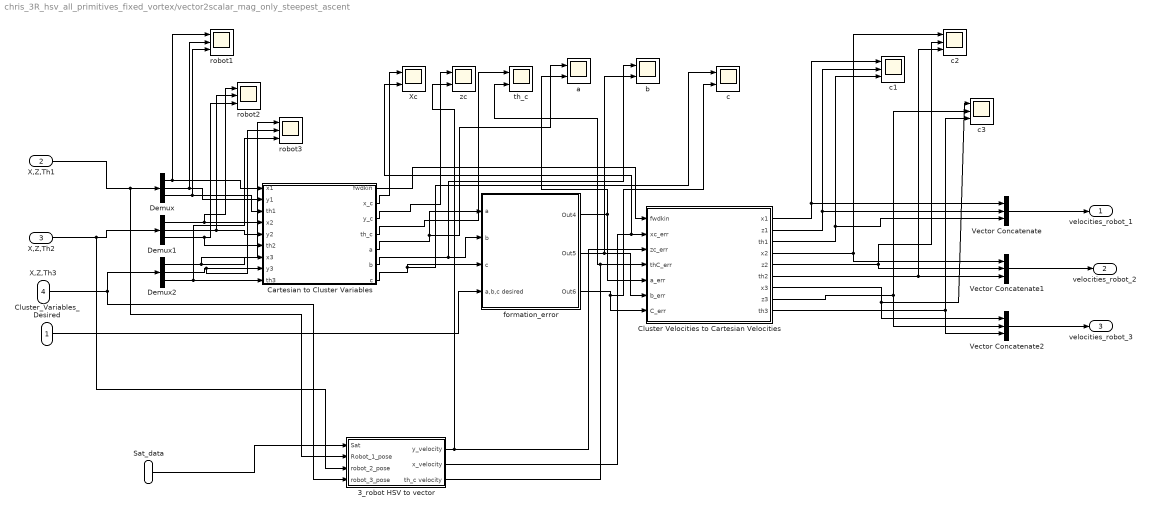
== system chris_3R_hsv_all_primitives_fixed_vortex/vector2scalar_mag_only_steepest_ascent ==
  Cluster_Variables_Desired : Inport
  X,Z,Th1 : Inport  Port=2
  X,Z,Th2 : Inport  Port=3
  X,Z,Th3 : Inport  Port=4
  Sat_data : Inport  Port=5
  3_robot HSV to vector : Subsystem
  Cartesian to Cluster Variables : MATLAB Function  TreatAsAtomicUnit=on
  Cluster Velocities to Cartesian Velocities : MATLAB Function  TreatAsAtomicUnit=on
  Demux : Demux  Outputs=3
  Demux1 : Demux  Outputs=3
  Demux2 : Demux  Outputs=3
  Vector Concatenate : Concatenate  NumInputs=3
  Vector Concatenate1 : Concatenate  NumInputs=3
  Vector Concatenate2 : Concatenate  NumInputs=3
  Xc : Scope  NumInputPorts=2
  a : Scope  NumInputPorts=2
  b : Scope  NumInputPorts=2
  c : Scope  NumInputPorts=2
  c1 : Scope  NumInputPorts=3
  c2 : Scope  NumInputPorts=3
  c3 : Scope  NumInputPorts=3
  formation_error : Subsystem
  robot1 : Scope  NumInputPorts=3
  robot2 : Scope  NumInputPorts=3
  robot3 : Scope  NumInputPorts=3
  th_c : Scope  NumInputPorts=2
  zc : Scope  NumInputPorts=2
  velocities_robot_1 : Outport
  velocities_robot_2 : Outport  Port=2
  velocities_robot_3 : Outport  Port=3
  wires:
  X,Z,Th1/1 -> 3_robot HSV to vector/2(Robot_1_pose), Demux/1
  X,Z,Th2/1 -> 3_robot HSV to vector/3(robot_2_pose), Demux1/1
  X,Z,Th3/1 -> Demux2/1, 3_robot HSV to vector/4(robot_3_pose)
  Vector Concatenate/1 -> velocities_robot_1/1
  Cluster Velocities to Cartesian Velocities/2(z1) -> c1/2, Vector Concatenate/2
  Cluster Velocities to Cartesian Velocities/1(x1) -> c1/1, Vector Concatenate/1
  Vector Concatenate1/1 -> velocities_robot_2/1
  Cluster Velocities to Cartesian Velocities/5(z2) -> c2/2, Vector Concatenate1/2
  Cluster Velocities to Cartesian Velocities/4(x2) -> c2/1, Vector Concatenate1/1
  Vector Concatenate2/1 -> velocities_robot_3/1
  Cluster Velocities to Cartesian Velocities/8(z3) -> c3/2, Vector Concatenate2/2
  Cluster Velocities to Cartesian Velocities/7(x3) -> Vector Concatenate2/1, c3/1
  Demux/1 -> robot1/1, Cartesian to Cluster Variables/1(x1)
  Demux/2 -> robot1/2, Cartesian to Cluster Variables/2(y1)
  Demux/3 -> robot1/3, Cartesian to Cluster Variables/3(th1)
  Demux1/1 -> robot2/1, Cartesian to Cluster Variables/4(x2)
  Demux1/2 -> robot2/2, Cartesian to Cluster Variables/5(y2)
  Demux1/3 -> robot2/3, Cartesian to Cluster Variables/6(th2)
  Demux2/1 -> robot3/1, Cartesian to Cluster Variables/7(x3)
  Demux2/2 -> robot3/2, Cartesian to Cluster Variables/8(y3)
  Demux2/3 -> robot3/3, Cartesian to Cluster Variables/9(th3)
  Cartesian to Cluster Variables/2(x_c) -> Xc/1
  Cartesian to Cluster Variables/3(y_c) -> zc/1
  Cartesian to Cluster Variables/4(th_c) -> th_c/1
  Cartesian to Cluster Variables/5(a) -> a/1, formation_error/1(a)
  Cartesian to Cluster Variables/6(b) -> b/1, formation_error/2(b)
  Cartesian to Cluster Variables/7(c) -> c/1, formation_error/3(c)
  Cluster_Variables_Desired/1 -> formation_error/4(a,b,c desired)
  formation_error/1(Out4) -> a/2, Cluster Velocities to Cartesian Velocities/5(a_err)
  formation_error/2(Out5) -> b/2, Cluster Velocities to Cartesian Velocities/6(b_err)
  formation_error/3(Out6) -> Cluster Velocities to Cartesian Velocities/7(C_err), c/2
  Cartesian to Cluster Variables/1(fwdkin) -> Cluster Velocities to Cartesian Velocities/1(fwdkin)
  Cluster Velocities to Cartesian Velocities/3(th1) -> c1/3, Vector Concatenate/3
  Cluster Velocities to Cartesian Velocities/6(th2) -> c2/3, Vector Concatenate1/3
  Cluster Velocities to Cartesian Velocities/9(th3) -> c3/3, Vector Concatenate2/3
  Sat_data/1 -> 3_robot HSV to vector/1(Sat)
  3_robot HSV to vector/2(x_velocity) -> Xc/2, Cluster Velocities to Cartesian Velocities/2(xc_err)
  3_robot HSV to vector/1(y_velocity) -> Cluster Velocities to Cartesian Velocities/3(zc_err), zc/2
  3_robot HSV to vector/3(th_c velocity) -> Cluster Velocities to Cartesian Velocities/4(thC_err), th_c/2

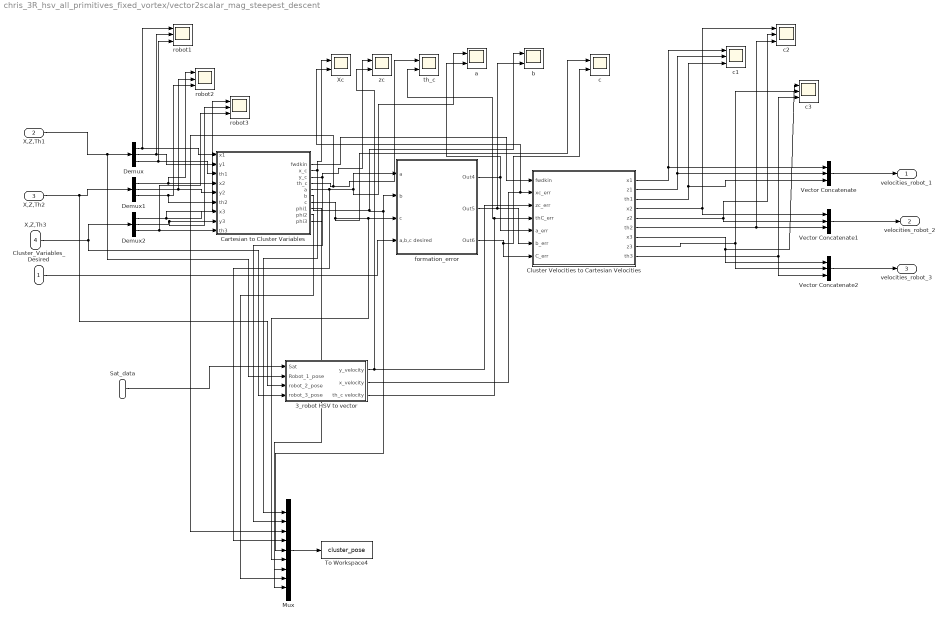
== system chris_3R_hsv_all_primitives_fixed_vortex/vector2scalar_mag_steepest_descent ==
  Cluster_Variables_Desired : Inport
  X,Z,Th1 : Inport  Port=2
  X,Z,Th2 : Inport  Port=3
  X,Z,Th3 : Inport  Port=4
  Sat_data : Inport  Port=5
  3_robot HSV to vector : Subsystem
  Cartesian to Cluster Variables : MATLAB Function  TreatAsAtomicUnit=on
  Cluster Velocities to Cartesian Velocities : MATLAB Function  TreatAsAtomicUnit=on
  Demux : Demux  Outputs=3
  Demux1 : Demux  Outputs=3
  Demux2 : Demux  Outputs=3
  Mux : Mux  Inputs=9
  To Workspace4 : ToWorkspace  VariableName=cluster_pose  SampleTime=-1
  Vector Concatenate : Concatenate  NumInputs=3
  Vector Concatenate1 : Concatenate  NumInputs=3
  Vector Concatenate2 : Concatenate  NumInputs=3
  Xc : Scope  NumInputPorts=2
  a : Scope  NumInputPorts=2
  b : Scope  NumInputPorts=2
  c : Scope  NumInputPorts=2
  c1 : Scope  NumInputPorts=3
  c2 : Scope  NumInputPorts=3
  c3 : Scope  NumInputPorts=3
  formation_error : Subsystem
  robot1 : Scope  NumInputPorts=3
  robot2 : Scope  NumInputPorts=3
  robot3 : Scope  NumInputPorts=3
  th_c : Scope  NumInputPorts=2
  zc : Scope  NumInputPorts=2
  velocities_robot_1 : Outport
  velocities_robot_2 : Outport  Port=2
  velocities_robot_3 : Outport  Port=3
  wires:
  X,Z,Th1/1 -> 3_robot HSV to vector/2(Robot_1_pose), Demux/1
  X,Z,Th2/1 -> 3_robot HSV to vector/3(robot_2_pose), Demux1/1
  X,Z,Th3/1 -> Demux2/1, 3_robot HSV to vector/4(robot_3_pose)
  Vector Concatenate/1 -> velocities_robot_1/1
  Cluster Velocities to Cartesian Velocities/2(z1) -> c1/2, Vector Concatenate/2
  Cluster Velocities to Cartesian Velocities/1(x1) -> c1/1, Vector Concatenate/1
  Vector Concatenate1/1 -> velocities_robot_2/1
  Cluster Velocities to Cartesian Velocities/5(z2) -> c2/2, Vector Concatenate1/2
  Cluster Velocities to Cartesian Velocities/4(x2) -> c2/1, Vector Concatenate1/1
  Vector Concatenate2/1 -> velocities_robot_3/1
  Cluster Velocities to Cartesian Velocities/8(z3) -> c3/2, Vector Concatenate2/2
  Cluster Velocities to Cartesian Velocities/7(x3) -> Vector Concatenate2/1, c3/1
  Demux/1 -> robot1/1, Cartesian to Cluster Variables/1(x1)
  Demux/2 -> robot1/2, Cartesian to Cluster Variables/2(y1)
  Demux/3 -> robot1/3, Cartesian to Cluster Variables/3(th1)
  Demux1/1 -> robot2/1, Cartesian to Cluster Variables/4(x2)
  Demux1/2 -> robot2/2, Cartesian to Cluster Variables/5(y2)
  Demux1/3 -> robot2/3, Cartesian to Cluster Variables/6(th2)
  Demux2/1 -> robot3/1, Cartesian to Cluster Variables/7(x3)
  Demux2/2 -> robot3/2, Cartesian to Cluster Variables/8(y3)
  Demux2/3 -> robot3/3, Cartesian to Cluster Variables/9(th3)
  Cartesian to Cluster Variables/2(x_c) -> Xc/1, Mux/1
  Cartesian to Cluster Variables/3(y_c) -> zc/1, Mux/2
  Cartesian to Cluster Variables/4(th_c) -> Mux/3, th_c/1
  Cartesian to Cluster Variables/5(a) -> a/1, formation_error/1(a), Mux/4
  Cartesian to Cluster Variables/6(b) -> formation_error/2(b), Mux/5, b/1
  Cartesian to Cluster Variables/7(c) -> c/1, Mux/6, formation_error/3(c)
  Cluster_Variables_Desired/1 -> formation_error/4(a,b,c desired)
  formation_error/1(Out4) -> a/2, Cluster Velocities to Cartesian Velocities/5(a_err)
  formation_error/2(Out5) -> b/2, Cluster Velocities to Cartesian Velocities/6(b_err)
  formation_error/3(Out6) -> Cluster Velocities to Cartesian Velocities/7(C_err), c/2
  Cartesian to Cluster Variables/1(fwdkin) -> Cluster Velocities to Cartesian Velocities/1(fwdkin)
  Cluster Velocities to Cartesian Velocities/3(th1) -> c1/3, Vector Concatenate/3
  Cluster Velocities to Cartesian Velocities/6(th2) -> c2/3, Vector Concatenate1/3
  Cluster Velocities to Cartesian Velocities/9(th3) -> c3/3, Vector Concatenate2/3
  Sat_data/1 -> 3_robot HSV to vector/1(Sat)
  3_robot HSV to vector/2(x_velocity) -> Xc/2, Cluster Velocities to Cartesian Velocities/2(xc_err)
  3_robot HSV to vector/1(y_velocity) -> Cluster Velocities to Cartesian Velocities/3(zc_err), zc/2
  3_robot HSV to vector/3(th_c velocity) -> Cluster Velocities to Cartesian Velocities/4(thC_err), th_c/2
  Mux/1 -> To Workspace4/1
  Cartesian to Cluster Variables/8(phi1) -> Mux/7
  Cartesian to Cluster Variables/9(phi2) -> Mux/8
  Cartesian to Cluster Variables/10(phi3) -> Mux/9

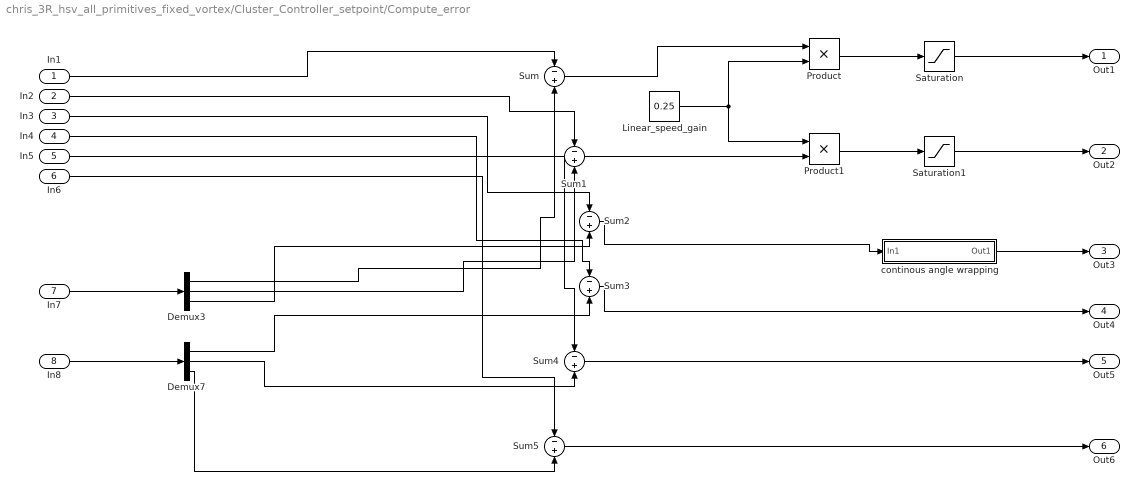
== system chris_3R_hsv_all_primitives_fixed_vortex/Cluster_Controller_setpoint/Compute_error ==
  In1 : Inport
  In2 : Inport  Port=2
  In3 : Inport  Port=3
  In4 : Inport  Port=4
  In5 : Inport  Port=5
  In6 : Inport  Port=6
  In7 : Inport  Port=7
  In8 : Inport  Port=8
  Demux3 : Demux  Outputs=3
  Demux7 : Demux  Outputs=3
  Linear_speed_gain : Constant  Value=0.25
  Product : Product
  Product1 : Product
  Saturation : Saturate
  Saturation1 : Saturate
  Sum{,1..5} (6 alike) : Sum  Inputs=-+
  continous angle wrapping : Subsystem
  Out1 : Outport
  Out2 : Outport  Port=2
  Out3 : Outport  Port=3
  Out4 : Outport  Port=4
  Out5 : Outport  Port=5
  Out6 : Outport  Port=6
  wires:
  In3/1 -> Sum2/1
  Demux3/2 -> Sum1/2
  Sum3/1 -> Out4/1
  In2/1 -> Sum1/1
  Demux3/3 -> Sum2/2
  Demux7/3 -> Sum5/2
  In8/1 -> Demux7/1
  Demux7/1 -> Sum3/2
  In1/1 -> Sum/1
  In5/1 -> Sum4/1
  Demux7/2 -> Sum4/2
  In6/1 -> Sum5/1
  Sum4/1 -> Out5/1
  Sum5/1 -> Out6/1
  Demux3/1 -> Sum/2
  In4/1 -> Sum3/1
  In7/1 -> Demux3/1
  Sum2/1 -> continous angle wrapping/1(In1)
  continous angle wrapping/1(Out1) -> Out3/1
  Sum/1 -> Product/1
  Linear_speed_gain/1 -> Product/2, Product1/1
  Sum1/1 -> Product1/2
  Saturation/1 -> Out1/1
  Product/1 -> Saturation/1
  Product1/1 -> Saturation1/1
  Saturation1/1 -> Out2/1
